simulink model "single_engine_neural_model_reference_control_learned_260120"  (R2018b)
settings: Solver=VariableStepAuto  StartTime=0.0  StopTime=10.0  RelTol=1e-3
libraries: neural x1
settings Model: Creator=Paweł Tymiński  LastModifiedBy=Paweł Tymiński

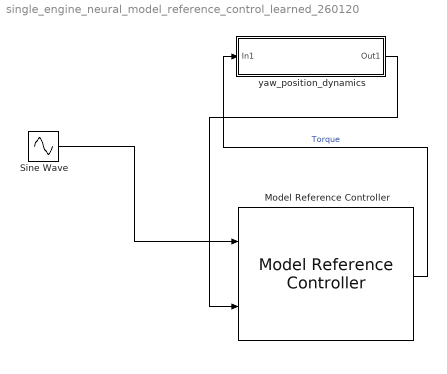
== system single_engine_neural_model_reference_control_learned_260120 ==
  Model Reference Controller : neural/Control Systems/Model Reference Controller  Nrc=1  Nic=1  Njc=1  IW_y=-0.0034933683544686308306  IW_u=0.0061154942035208104123  IW_r=0.0074297343432450334288  B1_c=-0.13251764525978854126  B2_c=12.75771057824404231  LW_c=96.848173048329940116  retraining_c=1  max_i_int=0.1  min_i_int=0.01  max_r_int=0.1  min_r_int=0.01  Ts=0.001  S1=1  Ni=1  Nj=1  sim_file=single_engine  trainfun=trainlm  Use_validation=1  Use_Testing=1  Use_Inc_training=0  Use_previous_weights=1  max_i=3  min_i=-3  max_r=3  min_r=-3  sam_training=1000  sam_training_c=1000  epochs=500  epochs_c=1000  minp=-2.7871332107799426936  maxp=2.7829416087142035963  mint=-2.7871332041362784082  maxt=2.7829416087142035963  Normalize=0  IW=0.030113674757846882468  LW1_2=0.084113124027856547849  LW2_1=9.0214635826486730963  B1=0.023955178600663540323  B2=-0.21458264600176421566  S1c=1  Limit_output=0  min_output=-Inf  max_output=Inf  Ref_file=single_engine
      settings: SourceProductName=Neural Network Toolbox  SourceProductBaseCode=NN
  Sine Wave : Sin  SampleTime=0
  yaw_position_dynamics : Subsystem
  wires:
  Model Reference Controller/1 -> yaw_position_dynamics/1(In1)  "Torque"
  yaw_position_dynamics/1(Out1) -> Model Reference Controller/2
  Sine Wave/1 -> Model Reference Controller/1

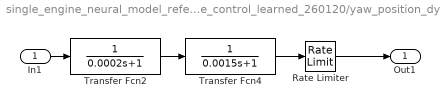
== system single_engine_neural_model_reference_control_learned_260120/yaw_position_dynamics ==
  In1 : Inport
  Rate Limiter : RateLimiter  RisingSlewLimit=18.5  FallingSlewLimit=-18.5  SampleTimeMode=inherited
  Transfer Fcn2 : TransferFcn  Denominator=[0.0002 1]
  Transfer Fcn4 : TransferFcn  Denominator=[0.0015 1]
  Out1 : Outport
  wires:
  Transfer Fcn2/1 -> Transfer Fcn4/1
  In1/1 -> Transfer Fcn2/1
  Transfer Fcn4/1 -> Rate Limiter/1
  Rate Limiter/1 -> Out1/1
